simulink model "arch_logical"  (R2024a)
settings: Solver=VariableStepAuto  StartTime=0.0  StopTime=2  RelTol=1e-3
model workspace (MAT data in the model file):
  Controller = Simulink.Parameter
  Controller.Value : enumeration (value not decoded)
  Controller.Complexity = 'real'
  Controller.Dimensions = [1 1]
  Controller.DataType = 'Enum: ControllerTypes'
  Controller.DocUnits = '1'
  obstacle_enable = Simulink.Parameter
  obstacle_enable.Value : enumeration (value not decoded)
  obstacle_enable.Complexity = 'real'
  obstacle_enable.Dimensions = [1 1]
  obstacle_enable.DataType = 'Enum: ObstacleMode'
  obstacle_enable.DocUnits = '1'
  pendulum_type = Simulink.Parameter
  pendulum_type.Value : enumeration (value not decoded)
  pendulum_type.Complexity = 'real'
  pendulum_type.Dimensions = [1 1]
  pendulum_type.DataType = 'Enum: PendulumTypes'
  pendulum_type.DocUnits = '1'
undefined symbols (not defined in the file): pendulum_mass, Ts
settings Model: DataDictionary=data_interface.sldd  Creator=upattacini  LastModifiedBy=amelis
settings DataIOCC: SaveOutput=off  DSMLogging=off  SaveTime=off  ReturnWorkspaceOutputs=off
settings ModelReferenceCC: ModelReferenceNumInstancesAllowed=Single
settings RTWCC: GPUComputeCapability=3.5
settings ExplorerConfigSet: SimMechanicsOpenEditorOnUpdate=off  InternalSimMechanicsExplorerSettings="<ExplorerConfiguration><canonicalview>default</canonicalview><AnimationSetting><BasePlaybackSpeed>1.0</BasePlaybackSpeed><PlaybackSpeedFactor>1.0</PlaybackSpeedFactor></AnimationSetting><TilePanel><TileInfo><Tiles Columns=\"1\" Count=\"1\" Rows=\"1\"><Column Weight=\"1\"/><Row Weight=\"1\"/><Tile Height=\"1\" Width=\"1\" X=\"0\" Y=\"0\"/></Tiles></TileInfo><SceneInfo><SceneViewer><BGColor><R>0.60000002384185791</R><G>0.60000002384185791</G><B>0.60000002384185791</B></BGColor><Camera><DoPerspective>off</DoPerspective><Position><X>-0.00879418750464690258</X><Y>0.0179244290375060247</Y><Z>1.00000000042813264</Z></Position><Center><X>-0.00879418750464690258</X><Y>0.0179244290375060247</Y><Z>4.28132640450940016e-10</Z></Center><Up><X>0</X><Y>1</Y><Z>-0</Z></Up><ViewLimDist>1</ViewLimDist><YLim>0.258153931099697476</YLim><XLim>0.345051321440949021</XLim></Camera></SceneViewer></SceneInfo></TilePanel><MechEditorPanel><Cameras/><GfxPanelCameraMap/><VideoCreator><PlaybackSpeedRatio>1.0</PlaybackSpeedRatio><FrameRate>30</FrameRate><VideoFormat>Motion JPEG AVI</VideoFormat><FrameSize>auto</FrameSize></VideoCreator></MechEditorPanel></ExplorerConfiguration>"

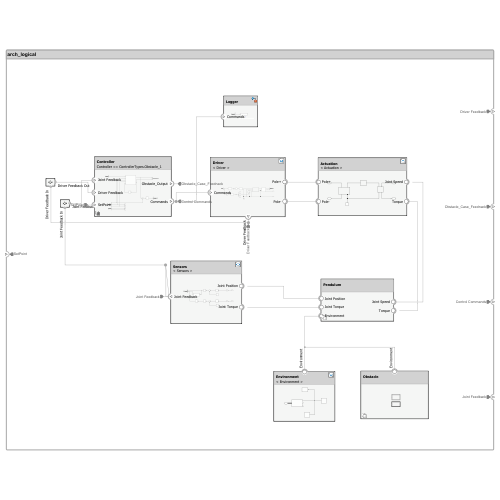
[thumbnail: Simulink's stored preview of the top-level diagram]
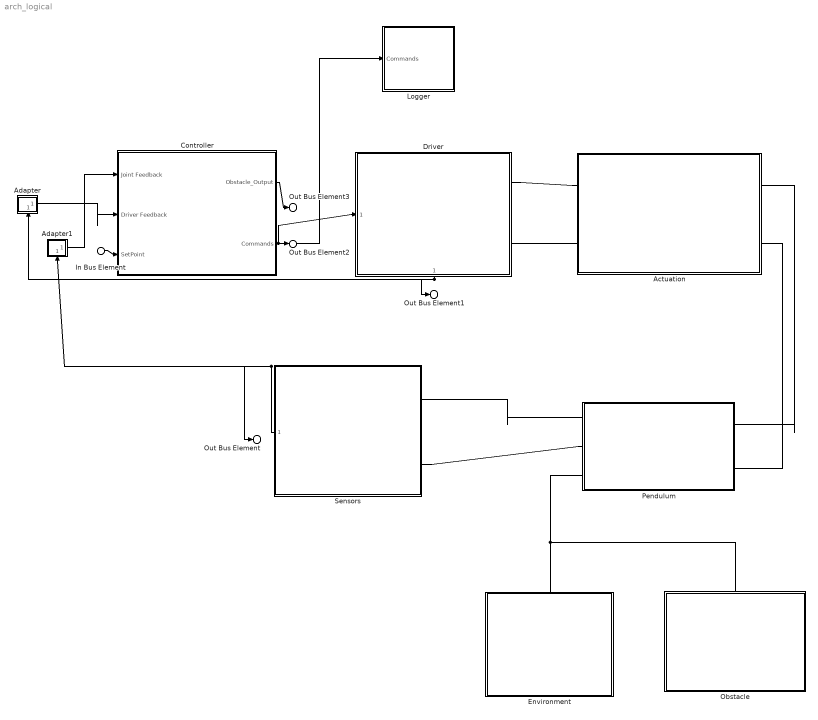
== system arch_logical ==
  In Bus Element : Inport  PortName=SetPoint
  Actuation : Subsystem  ReferencedSubsystem=Actuation
      settings: PermitHierarchicalResolution=None  PortSchema="{\"entries\":[{\"content\":{\"headerSize\":26,\"margin\":15,\"minimumSpacing\":25,\"sides\":[{\"content\":{\"connectorIds\":[\"LConn1\",\"LConn2\"]},\"type\":\"ConnectorPlacement.EquallySpacedRectSide\",\"uuid\":\"cda6e8c3-28ef-478a-8903-19efeda1d005\"},{\"content\":{\"connectorIds\":[\"RConn1\",\"RConn2\"],\"side\":\"RIGHT\"},\"type\":\"ConnectorPlacement.EquallySpacedRectSide\",\"uuid\":\"ea374fb9-fe28-40dc-ac3e-322c9df25f40\"},{\"content\":{\"side\":\"TOP\"},\"type\":\"ConnectorPlacement.EquallySpacedRectSide\",\"uuid\":\"d8bce015-985d-440b-ab42-a24854ac657a\"}]},\"type\":\"ConnectorPlacement.EquallySpacedConnector\",\"uuid\":\"3fae5f3d-400e-4110-946e-917d26d89769\"}],\"packageUris\":[\"http://schema.mathworks.com/mf0/Connector/R2020b\"],\"version\":\"1.0\"}"
  Adapter : Subsystem
      settings: PortSchema="{\"entries\":[{\"content\":{\"margin\":10,\"minimumSpacing\":15,\"sides\":[{\"content\":{},\"type\":\"ConnectorPlacement.EquallySpacedRectSide\",\"uuid\":\"71c09ee4-bd5d-4849-9770-0bb167b66dd4\"},{\"content\":{\"connectorIds\":[\"Out1\"],\"side\":\"RIGHT\"},\"type\":\"ConnectorPlacement.EquallySpacedRectSide\",\"uuid\":\"3c6482b7-7dc2-4555-8349-1ada307188c7\"},{\"content\":{\"side\":\"TOP\"},\"type\":\"ConnectorPlacement.EquallySpacedRectSide\",\"uuid\":\"1ceef67c-8610-4005-8087-2f0234552c2e\"},{\"content\":{\"connectorIds\":[\"In1\"],\"side\":\"BOTTOM\"},\"type\":\"ConnectorPlacement.EquallySpacedRectSide\",\"uuid\":\"af19ee06-0b8c-42bc-982e-14fd9028925b\"}]},\"type\":\"ConnectorPlacement.EquallySpacedConnector\",\"uuid\":\"27bb57db-ed53-47ec-ba16-e40a00874efd\"}],\"packageUris\":[\"http://schema.mathworks.com/mf0/Connector/R2020b\"],\"version\":\"1.0\"}"
  Adapter1 : Subsystem
      settings: PortSchema="{\"entries\":[{\"content\":{\"margin\":10,\"minimumSpacing\":15,\"sides\":[{\"content\":{},\"type\":\"ConnectorPlacement.EquallySpacedRectSide\",\"uuid\":\"7b1645bb-00f8-429a-b5aa-c1090bce1ac1\"},{\"content\":{\"connectorIds\":[\"Out1\"],\"side\":\"RIGHT\"},\"type\":\"ConnectorPlacement.EquallySpacedRectSide\",\"uuid\":\"0ba1b368-e635-485c-8963-63f2d5c928f2\"},{\"content\":{\"side\":\"TOP\"},\"type\":\"ConnectorPlacement.EquallySpacedRectSide\",\"uuid\":\"b189292e-591f-40ba-a07d-c96754195ee8\"},{\"content\":{\"connectorIds\":[\"In1\"],\"side\":\"BOTTOM\"},\"type\":\"ConnectorPlacement.EquallySpacedRectSide\",\"uuid\":\"9572e0d9-6fe3-42e3-bf06-cb923272bc1d\"}]},\"type\":\"ConnectorPlacement.EquallySpacedConnector\",\"uuid\":\"d599bba2-5016-4d49-948e-964efe72a785\"}],\"packageUris\":[\"http://schema.mathworks.com/mf0/Connector/R2020b\"],\"version\":\"1.0\"}"
  Controller : Subsystem  Variant=on  VariantControlMode=label  VariantControl=Controller  LabelModeActiveChoice=Controller == ControllerTypes.Obstacle_1
      settings: PortSchema="{\"entries\":[{\"content\":{\"headerSize\":38,\"margin\":15,\"minimumSpacing\":25,\"sides\":[{\"content\":{\"connectorIds\":[\"In3\",\"In1\",\"In2\"]},\"type\":\"ConnectorPlacement.EquallySpacedRectSide\",\"uuid\":\"cda6e8c3-28ef-478a-8903-19efeda1d005\"},{\"content\":{\"connectorIds\":[\"Out1\",\"Out2\"],\"side\":\"RIGHT\"},\"type\":\"ConnectorPlacement.EquallySpacedRectSide\",\"uuid\":\"ea374fb9-fe28-40dc-ac3e-322c9df25f40\"},{\"content\":{\"side\":\"TOP\"},\"type\":\"ConnectorPlacement.EquallySpacedRectSide\",\"uuid\":\"d8bce015-985d-440b-ab42-a24854ac657a\"},{\"content\":{\"side\":\"BOTTOM\"},\"type\":\"ConnectorPlacement.EquallySpacedRectSide\",\"uuid\":\"ef4904ce-87a8-4dd7-afa5-50688cfaf5d0\"}]},\"type\":\"ConnectorPlacement.EquallySpacedConnector\",\"uuid\":\"3fae5f3d-400e-4110-946e-917d26d89769\"}],\"packageUris\":[\"http://schema.mathworks.com/mf0/Connector/R2020b\"],\"version\":\"1.0\"}"
  Driver : Subsystem  ReferencedSubsystem=Driver
      settings: PermitHierarchicalResolution=None  PortSchema="{\"entries\":[{\"content\":{\"headerSize\":26,\"margin\":15,\"minimumSpacing\":25,\"sides\":[{\"content\":{\"connectorIds\":[\"In1\"]},\"type\":\"ConnectorPlacement.EquallySpacedRectSide\",\"uuid\":\"87b13320-d2be-495c-9e0a-d50be08d4455\"},{\"content\":{\"connectorIds\":[\"RConn1\",\"RConn2\"],\"side\":\"RIGHT\"},\"type\":\"ConnectorPlacement.EquallySpacedRectSide\",\"uuid\":\"602bd151-4107-439e-8200-46b9490e5c42\"},{\"content\":{\"side\":\"TOP\"},\"type\":\"ConnectorPlacement.EquallySpacedRectSide\",\"uuid\":\"a9c961f8-1e8e-4fd0-91ed-15da0975152b\"},{\"content\":{\"connectorIds\":[\"Out1\"],\"side\":\"BOTTOM\"},\"type\":\"ConnectorPlacement.EquallySpacedRectSide\",\"uuid\":\"ffc1b1ec-88d8-4f39-9e46-3aab7c832f5b\"}]},\"type\":\"ConnectorPlacement.EquallySpacedConnector\",\"uuid\":\"8c5d9a44-25d8-4d3b-8680-514fbe3d26a8\"}],\"packageUris\":[\"http://schema.mathworks.com/mf0/Connector/R2020b\"],\"version\":\"1.0\"}"
  Environment : Subsystem  ReferencedSubsystem=Environment
      settings: PermitHierarchicalResolution=None  PortSchema="{\"entries\":[{\"content\":{\"headerSize\":26,\"margin\":15,\"minimumSpacing\":25,\"sides\":[{\"content\":{},\"type\":\"ConnectorPlacement.EquallySpacedRectSide\",\"uuid\":\"45a2255a-b64b-4ce6-b48f-d923e11d651c\"},{\"content\":{\"side\":\"RIGHT\"},\"type\":\"ConnectorPlacement.EquallySpacedRectSide\",\"uuid\":\"23c27b1d-8e45-436e-af19-695457c59d8d\"},{\"content\":{\"connectorIds\":[\"LConn1\"],\"side\":\"TOP\"},\"type\":\"ConnectorPlacement.EquallySpacedRectSide\",\"uuid\":\"da7f94f3-b927-4bf7-a124-148f2fc7ec34\"}]},\"type\":\"ConnectorPlacement.EquallySpacedConnector\",\"uuid\":\"db435fa4-4dbe-4289-bd60-c3db6d84fa67\"}],\"packageUris\":[\"http://schema.mathworks.com/mf0/Connector/R2020b\"],\"version\":\"1.0\"}"
  Logger : Subsystem
      settings: PortSchema="{\"entries\":[{\"content\":{\"headerSize\":26,\"margin\":15,\"minimumSpacing\":25,\"sides\":[{\"content\":{\"connectorIds\":[\"In1\"]},\"type\":\"ConnectorPlacement.EquallySpacedRectSide\",\"uuid\":\"ac000ab5-2ae6-4b56-9db1-279b30760399\"},{\"content\":{\"side\":\"RIGHT\"},\"type\":\"ConnectorPlacement.EquallySpacedRectSide\",\"uuid\":\"5b386faf-72fc-41cd-a667-c083d520b36c\"},{\"content\":{\"side\":\"TOP\"},\"type\":\"ConnectorPlacement.EquallySpacedRectSide\",\"uuid\":\"dd48b8b5-1971-43a9-94c4-f2d4d7fadaf4\"}]},\"type\":\"ConnectorPlacement.EquallySpacedConnector\",\"uuid\":\"b0312a47-d361-4d2b-90c8-709d42774a27\"}],\"packageUris\":[\"http://schema.mathworks.com/mf0/Connector/R2020b\"],\"version\":\"1.0\"}"
  Obstacle : Subsystem  Variant=on
      settings: PortSchema="{\"entries\":[{\"content\":{\"headerSize\":38,\"margin\":15,\"minimumSpacing\":25,\"sides\":[{\"content\":{},\"type\":\"ConnectorPlacement.EquallySpacedRectSide\",\"uuid\":\"af0407ec-1779-49f3-b108-c3c3f6f7c598\"},{\"content\":{\"side\":\"RIGHT\"},\"type\":\"ConnectorPlacement.EquallySpacedRectSide\",\"uuid\":\"b7d68d59-9a8d-4e89-bbf6-2538cb959734\"},{\"content\":{\"connectorIds\":[\"LConn1\"],\"side\":\"TOP\"},\"type\":\"ConnectorPlacement.EquallySpacedRectSide\",\"uuid\":\"a81bca48-206b-4df8-8ce5-894836e99913\"}]},\"type\":\"ConnectorPlacement.EquallySpacedConnector\",\"uuid\":\"b741c75d-e85b-44d8-8ecc-6dd0b77ab435\"}],\"packageUris\":[\"http://schema.mathworks.com/mf0/Connector/R2020b\"],\"version\":\"1.0\"}"
  Pendulum : Subsystem  Variant=on
      settings: PortSchema="{\"entries\":[{\"content\":{\"headerSize\":38,\"margin\":15,\"minimumSpacing\":25,\"sides\":[{\"content\":{\"connectorIds\":[\"LConn2\",\"LConn3\",\"LConn1\"]},\"type\":\"ConnectorPlacement.EquallySpacedRectSide\",\"uuid\":\"bf58af0e-2227-4325-b7b4-ca7aa5d9b389\"},{\"content\":{\"connectorIds\":[\"RConn1\",\"RConn2\"],\"side\":\"RIGHT\"},\"type\":\"ConnectorPlacement.EquallySpacedRectSide\",\"uuid\":\"91e52710-35d3-4d9b-803d-8a6447c25190\"},{\"content\":{\"side\":\"TOP\"},\"type\":\"ConnectorPlacement.EquallySpacedRectSide\",\"uuid\":\"a9a735dd-f81f-408b-81bc-2d8dc361c4fb\"}]},\"type\":\"ConnectorPlacement.EquallySpacedConnector\",\"uuid\":\"4c4e0bb0-440d-47ff-82c5-294788dc91eb\"}],\"packageUris\":[\"http://schema.mathworks.com/mf0/Connector/R2020b\"],\"version\":\"1.0\"}"
  Sensors : Subsystem  ReferencedSubsystem=Sensors
      settings: PermitHierarchicalResolution=None  PortSchema="{\"entries\":[{\"content\":{\"headerSize\":26,\"margin\":15,\"minimumSpacing\":25,\"sides\":[{\"content\":{\"connectorIds\":[\"Out1\"]},\"type\":\"ConnectorPlacement.EquallySpacedRectSide\",\"uuid\":\"45a2255a-b64b-4ce6-b48f-d923e11d651c\"},{\"content\":{\"connectorIds\":[\"RConn1\",\"RConn2\"],\"side\":\"RIGHT\"},\"type\":\"ConnectorPlacement.EquallySpacedRectSide\",\"uuid\":\"23c27b1d-8e45-436e-af19-695457c59d8d\"},{\"content\":{\"side\":\"TOP\"},\"type\":\"ConnectorPlacement.EquallySpacedRectSide\",\"uuid\":\"da7f94f3-b927-4bf7-a124-148f2fc7ec34\"}]},\"type\":\"ConnectorPlacement.EquallySpacedConnector\",\"uuid\":\"db435fa4-4dbe-4289-bd60-c3db6d84fa67\"}],\"packageUris\":[\"http://schema.mathworks.com/mf0/Connector/R2020b\"],\"version\":\"1.0\"}"
  Out Bus Element1 : Outport  PortName=Driver Feedback
  Out Bus Element3 : Outport  Port=2  PortName=Obstacle_Case_Feednack
  Out Bus Element2 : Outport  Port=3  PortName=Control Commands
  Out Bus Element : Outport  Port=4  PortName=Joint Feedback
  wires:
  Driver/1 -> Out Bus Element1/1, Adapter/1(Driver Feedback In)
  Sensors/1 -> Out Bus Element/1, Adapter1/1(Joint Feedback In)
  In Bus Element/1 -> Controller/2(SetPoint)
  Adapter1/1(Joint Feedback Out) -> Controller/3(Joint Feedback)
  Adapter/1(Driver Feedback Out) -> Controller/1(Driver Feedback)
  Controller/2(Commands) -> Logger/1(Commands), Out Bus Element2/1, Driver/1
  Controller/1(Obstacle_Output) -> Out Bus Element3/1
  connections:
  Environment/LConn1 -- Pendulum/LConn1 -- Obstacle/LConn1
  Sensors/RConn1 -- Pendulum/LConn2
  Sensors/RConn2 -- Pendulum/LConn3
  Driver/RConn1 -- Actuation/LConn1
  Driver/RConn2 -- Actuation/LConn2
  Actuation/RConn1 -- Pendulum/RConn1
  Actuation/RConn2 -- Pendulum/RConn2

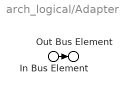
== system arch_logical/Adapter ==
  In Bus Element : Inport  PortName=Driver Feedback In
  Out Bus Element : Outport  PortName=Driver Feedback Out
  wires:
  In Bus Element/1 -> Out Bus Element/1

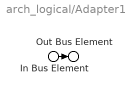
== system arch_logical/Adapter1 ==
  In Bus Element : Inport  PortName=Joint Feedback In
  Out Bus Element : Outport  PortName=Joint Feedback Out
  wires:
  In Bus Element/1 -> Out Bus Element/1

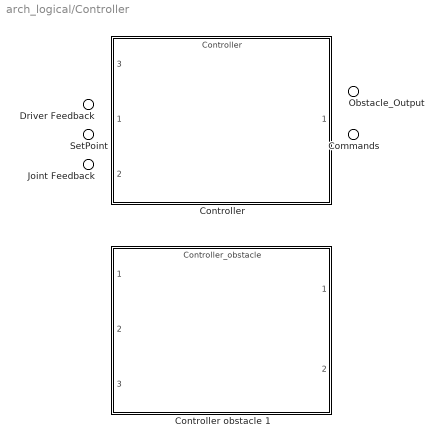
== system arch_logical/Controller ==
  Driver Feedback : Inport
  SetPoint : Inport  Port=2
  Joint Feedback : Inport  Port=3
  Controller : ModelReference  ModelNameDialog=Controller  SimulationMode=Normal  VariantControl=Controller == ControllerTypes.Basic  ModelReferenceVersion=2.120
      settings: PortSchema="{\"entries\":[{\"content\":{\"headerSize\":38,\"margin\":15,\"minimumSpacing\":25,\"sides\":[{\"content\":{\"connectorIds\":[\"In3\",\"In1\",\"In2\"]},\"type\":\"ConnectorPlacement.EquallySpacedRectSide\",\"uuid\":\"cda6e8c3-28ef-478a-8903-19efeda1d005\"},{\"content\":{\"connectorIds\":[\"Out1\"],\"side\":\"RIGHT\"},\"type\":\"ConnectorPlacement.EquallySpacedRectSide\",\"uuid\":\"ea374fb9-fe28-40dc-ac3e-322c9df25f40\"},{\"content\":{\"side\":\"TOP\"},\"type\":\"ConnectorPlacement.EquallySpacedRectSide\",\"uuid\":\"d8bce015-985d-440b-ab42-a24854ac657a\"},{\"content\":{\"side\":\"BOTTOM\"},\"type\":\"ConnectorPlacement.EquallySpacedRectSide\",\"uuid\":\"ef4904ce-87a8-4dd7-afa5-50688cfaf5d0\"}]},\"type\":\"ConnectorPlacement.EquallySpacedConnector\",\"uuid\":\"3fae5f3d-400e-4110-946e-917d26d89769\"}],\"packageUris\":[\"http://schema.mathworks.com/mf0/Connector/R2020b\"],\"version\":\"1.0\"}"
  Controller obstacle 1 : ModelReference  ModelNameDialog=Controller_obstacle  SimulationMode=Normal  VariantControl=Controller == ControllerTypes.Obstacle_1  ModelReferenceVersion=2.118
      settings: PortSchema="{\"entries\":[{\"content\":{\"headerSize\":38,\"margin\":15,\"minimumSpacing\":25,\"sides\":[{\"content\":{\"connectorIds\":[\"In1\",\"In2\",\"In3\"]},\"type\":\"ConnectorPlacement.EquallySpacedRectSide\",\"uuid\":\"cda6e8c3-28ef-478a-8903-19efeda1d005\"},{\"content\":{\"connectorIds\":[\"Out1\",\"Out2\"],\"side\":\"RIGHT\"},\"type\":\"ConnectorPlacement.EquallySpacedRectSide\",\"uuid\":\"ea374fb9-fe28-40dc-ac3e-322c9df25f40\"},{\"content\":{\"side\":\"TOP\"},\"type\":\"ConnectorPlacement.EquallySpacedRectSide\",\"uuid\":\"d8bce015-985d-440b-ab42-a24854ac657a\"},{\"content\":{\"side\":\"BOTTOM\"},\"type\":\"ConnectorPlacement.EquallySpacedRectSide\",\"uuid\":\"ef4904ce-87a8-4dd7-afa5-50688cfaf5d0\"}]},\"type\":\"ConnectorPlacement.EquallySpacedConnector\",\"uuid\":\"3fae5f3d-400e-4110-946e-917d26d89769\"}],\"packageUris\":[\"http://schema.mathworks.com/mf0/Connector/R2020b\"],\"version\":\"1.0\"}"
  Obstacle_Output : Outport  OutDataTypeStr=Bus: Obstacle_Case_Feedback
  Commands : Outport  Port=2

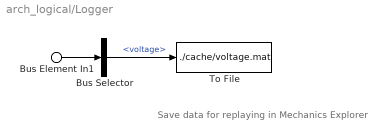
== system arch_logical/Logger ==
  note: Save data for replaying in Mechanics Explorer
  Bus Element In1 : Inport  PortName=Commands
  Bus Selector : BusSelector  OutputSignals=voltage
  To File : ToFile  Filename=./cache/voltage.mat  MatrixName=voltage  SaveFormat=Timeseries  SampleTime=Ts
  wires:
  Bus Selector/1 -> To File/1  "<voltage>"
  Bus Element In1/1 -> Bus Selector/1

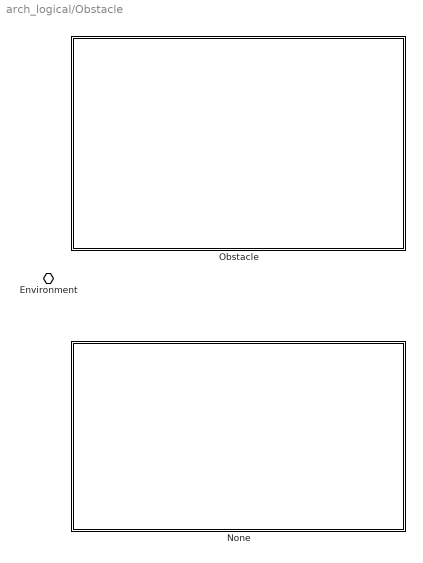
== system arch_logical/Obstacle ==
  None : Subsystem  VariantControl=obstacle_enable == ObstacleMode.Off
      settings: PortSchema="{\"entries\":[{\"content\":{\"headerSize\":26,\"margin\":15,\"minimumSpacing\":25,\"sides\":[{\"content\":{\"connectorIds\":[\"LConn1\"]},\"type\":\"ConnectorPlacement.EquallySpacedRectSide\",\"uuid\":\"0a5e0032-de0c-4e65-8963-45a8180f174e\"},{\"content\":{\"side\":\"RIGHT\"},\"type\":\"ConnectorPlacement.EquallySpacedRectSide\",\"uuid\":\"c045804f-1e8f-41b0-95f9-8d38ee90510b\"},{\"content\":{\"side\":\"TOP\"},\"type\":\"ConnectorPlacement.EquallySpacedRectSide\",\"uuid\":\"a5646e63-3654-4592-b7ee-151ade11516d\"}]},\"type\":\"ConnectorPlacement.EquallySpacedConnector\",\"uuid\":\"d901f530-b744-4bfb-8642-2cc9145429f9\"}],\"packageUris\":[\"http://schema.mathworks.com/mf0/Connector/R2020b\"],\"version\":\"1.0\"}"
  Obstacle : Subsystem  VariantControl=obstacle_enable == ObstacleMode.On  ReferencedSubsystem=Obstacle  l=0.5  m=0.1
      settings: PermitHierarchicalResolution=None  PortSchema="{\"entries\":[{\"content\":{\"headerSize\":26,\"margin\":15,\"minimumSpacing\":25,\"sides\":[{\"content\":{\"connectorIds\":[\"LConn1\"]},\"type\":\"ConnectorPlacement.EquallySpacedRectSide\",\"uuid\":\"0a5e0032-de0c-4e65-8963-45a8180f174e\"},{\"content\":{\"side\":\"RIGHT\"},\"type\":\"ConnectorPlacement.EquallySpacedRectSide\",\"uuid\":\"c045804f-1e8f-41b0-95f9-8d38ee90510b\"},{\"content\":{\"side\":\"TOP\"},\"type\":\"ConnectorPlacement.EquallySpacedRectSide\",\"uuid\":\"a5646e63-3654-4592-b7ee-151ade11516d\"}]},\"type\":\"ConnectorPlacement.EquallySpacedConnector\",\"uuid\":\"d901f530-b744-4bfb-8642-2cc9145429f9\"}],\"packageUris\":[\"http://schema.mathworks.com/mf0/Connector/R2020b\"],\"version\":\"1.0\"}"
  Environment : PMIOPort  Side=Left

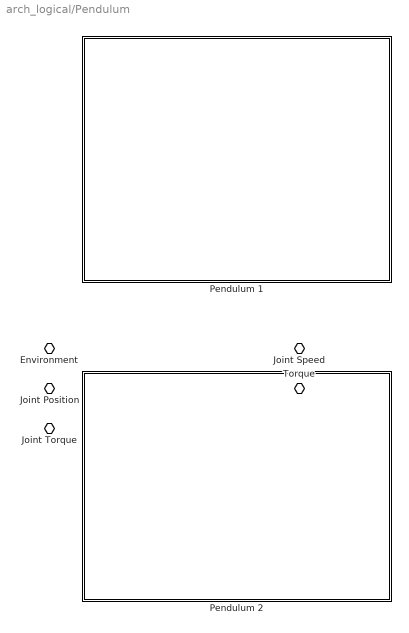
== system arch_logical/Pendulum ==
  Pendulum 1 : Subsystem  VariantControl=pendulum_type == PendulumTypes.Pendulum_1  ReferencedSubsystem=Pendulum  l=pendulum_1_length  m=pendulum_mass
      settings: PermitHierarchicalResolution=None  PortSchema="{\"entries\":[{\"content\":{\"headerSize\":26,\"margin\":15,\"minimumSpacing\":25,\"sides\":[{\"content\":{\"connectorIds\":[\"LConn1\",\"LConn2\",\"LConn3\"]},\"type\":\"ConnectorPlacement.EquallySpacedRectSide\",\"uuid\":\"82f5cb4d-4a78-40c4-a21e-410695f42653\"},{\"content\":{\"connectorIds\":[\"RConn1\",\"RConn2\"],\"side\":\"RIGHT\"},\"type\":\"ConnectorPlacement.EquallySpacedRectSide\",\"uuid\":\"035de433-2e3e-4321-a7d9-a74f0d831365\"},{\"content\":{\"side\":\"TOP\"},\"type\":\"ConnectorPlacement.EquallySpacedRectSide\",\"uuid\":\"ce921c4a-a98b-4acd-b6b2-e0e0d1283243\"}]},\"type\":\"ConnectorPlacement.EquallySpacedConnector\",\"uuid\":\"03220c26-1eff-4576-b7d6-6d5cd293b475\"}],\"packageUris\":[\"http://schema.mathworks.com/mf0/Connector/R2020b\"],\"version\":\"1.0\"}"
  Pendulum 2 : Subsystem  VariantControl=pendulum_type == PendulumTypes.Pendulum_2  ReferencedSubsystem=Pendulum  l=pendulum_2_length  m=pendulum_mass
      settings: PermitHierarchicalResolution=None  PortSchema="{\"entries\":[{\"content\":{\"headerSize\":26,\"margin\":15,\"minimumSpacing\":25,\"sides\":[{\"content\":{\"connectorIds\":[\"LConn1\",\"LConn2\",\"LConn3\"]},\"type\":\"ConnectorPlacement.EquallySpacedRectSide\",\"uuid\":\"82f5cb4d-4a78-40c4-a21e-410695f42653\"},{\"content\":{\"connectorIds\":[\"RConn1\",\"RConn2\"],\"side\":\"RIGHT\"},\"type\":\"ConnectorPlacement.EquallySpacedRectSide\",\"uuid\":\"035de433-2e3e-4321-a7d9-a74f0d831365\"},{\"content\":{\"side\":\"TOP\"},\"type\":\"ConnectorPlacement.EquallySpacedRectSide\",\"uuid\":\"ce921c4a-a98b-4acd-b6b2-e0e0d1283243\"}]},\"type\":\"ConnectorPlacement.EquallySpacedConnector\",\"uuid\":\"03220c26-1eff-4576-b7d6-6d5cd293b475\"}],\"packageUris\":[\"http://schema.mathworks.com/mf0/Connector/R2020b\"],\"version\":\"1.0\"}"
  Joint Speed : PMIOPort  Side=Right
  Torque : PMIOPort  Port=2  Side=Right
  Environment : PMIOPort  Port=3  Side=Left
  Joint Position : PMIOPort  Port=4  Side=Left
  Joint Torque : PMIOPort  Port=5  Side=Left

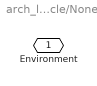
== system arch_logical/Obstacle/None ==
  Environment : PMIOPort  Side=Left
